simulink model "EV_assigment2"  (R2022a)
settings: Solver=VariableStepAuto  StartTime=0.0  StopTime=10800  RelTol=1e-3
libraries: spsCurrentMeasurementLib x141, spsSeriesRLCBranchLib x141, spsVoltageMeasurementLib x141, spsControlledVoltageSourceLib x140, spspowerguiLib x1
(part 3 of 15)

== system EV_assigment2/series1/Subsystem19 ==
  Controlled Voltage Source : spsControlledVoltageSourceLib/Controlled Voltage Source  Initialize=on  Source_Type=AC  Amplitude=0  Phase=0  Frequency=0  Measurements=None
  Current Measurement : spsCurrentMeasurementLib/Current Measurement  PhasorSimulation=off  OutputType=Complex  PSBequivalent=0
  Display : Display
  Display1 : Display
  Divide1 : Product  Inputs=*/
  Divide2 : Product  Inputs=*//
  Initial Capacity(Ah) : Constant  Value=28
  Integrator Limited : Integrator  LimitOutput=on  UpperSaturationLimit=1  LowerSaturationLimit=0
  LoadAh : Scope
  Product : Product
  SOC : Scope
  SOC value : Display
  Scope : Scope
  Scope1 : Scope
  Series RLC Branch : spsSeriesRLCBranchLib/Series RLC Branch  LConnTagsString=__new0  RConnTagsString=__new0  BranchType=R  Resistance=1e-6  Inductance=1e-3  SetiL0=off  InitialCurrent=0  Capacitance=1e-6  Setx0=off  InitialVoltage=0  Measurements=None
  Subsystem : Subsystem
  Subsystem1 : Subsystem
  Sum : Sum  Inputs=|+-
  Sum1 : Sum  Inputs=+--
  Voltage Measurement : spsVoltageMeasurementLib/Voltage Measurement  PhasorSimulation=off  OutputType=Complex  PSBequivalent=0
  battery Temp(k) : Constant  Value=300
  + : PMIOPort  Side=Left
  - : PMIOPort  Port=2  Side=Right
  wires:
  Subsystem/3(R1) -> Divide2/2
  Divide1/1 -> Sum/1
  Product/1 -> Sum1/2
  Current Measurement/1 -> Display1/1, Scope/1, Divide1/1, Product/2, Subsystem1/1(Battery Current)
  Subsystem/1(Em) -> Sum1/1
  battery Temp(k)/1 -> Subsystem1/3(Temp(K)), Subsystem/2(Battery temp)
  Sum/1 -> Integrator Limited/1
  Divide2/1 -> Sum/2
  Subsystem/2(R0) -> Product/1
  Integrator Limited/1 -> Divide2/1, Sum1/3
  Subsystem/4(C1) -> Divide2/3, Divide1/2
  Sum1/1 -> Controlled Voltage Source/1
  Subsystem1/2(SOC) -> Subsystem/1(SOC), SOC value/1, SOC/1
  Subsystem1/1(LoadAh) -> LoadAh/1
  Initial Capacity(Ah)/1 -> Subsystem1/2(InitCap(Ah))
  Voltage Measurement/1 -> Display/1, Scope1/1
  connections:
  Series RLC Branch/RConn1 -- Voltage Measurement/LConn1 -- Current Measurement/LConn1
  Current Measurement/RConn1 -- +/RConn1
  Controlled Voltage Source/LConn1 -- Voltage Measurement/LConn2 -- -/RConn1
  Series RLC Branch/LConn1 -- Controlled Voltage Source/RConn1

== system EV_assigment2/series1/Subsystem2 ==
  Controlled Voltage Source : spsControlledVoltageSourceLib/Controlled Voltage Source  Initialize=on  Source_Type=AC  Amplitude=0  Phase=0  Frequency=0  Measurements=None
  Current Measurement : spsCurrentMeasurementLib/Current Measurement  PhasorSimulation=off  OutputType=Complex  PSBequivalent=0
  Display : Display
  Display1 : Display
  Divide1 : Product  Inputs=*/
  Divide2 : Product  Inputs=*//
  Initial Capacity(Ah) : Constant  Value=28
  Integrator Limited : Integrator  LimitOutput=on  UpperSaturationLimit=1  LowerSaturationLimit=0
  LoadAh : Scope
  Product : Product
  SOC : Scope
  SOC value : Display
  Scope : Scope
  Scope1 : Scope
  Series RLC Branch : spsSeriesRLCBranchLib/Series RLC Branch  LConnTagsString=__new0  RConnTagsString=__new0  BranchType=R  Resistance=1e-6  Inductance=1e-3  SetiL0=off  InitialCurrent=0  Capacitance=1e-6  Setx0=off  InitialVoltage=0  Measurements=None
  Subsystem : Subsystem
  Subsystem1 : Subsystem
  Sum : Sum  Inputs=|+-
  Sum1 : Sum  Inputs=+--
  Voltage Measurement : spsVoltageMeasurementLib/Voltage Measurement  PhasorSimulation=off  OutputType=Complex  PSBequivalent=0
  battery Temp(k) : Constant  Value=300
  + : PMIOPort  Side=Left
  - : PMIOPort  Port=2  Side=Right
  wires:
  Subsystem/3(R1) -> Divide2/2
  Divide1/1 -> Sum/1
  Product/1 -> Sum1/2
  Current Measurement/1 -> Display1/1, Scope/1, Divide1/1, Product/2, Subsystem1/1(Battery Current)
  Subsystem/1(Em) -> Sum1/1
  battery Temp(k)/1 -> Subsystem1/3(Temp(K)), Subsystem/2(Battery temp)
  Sum/1 -> Integrator Limited/1
  Divide2/1 -> Sum/2
  Subsystem/2(R0) -> Product/1
  Integrator Limited/1 -> Divide2/1, Sum1/3
  Subsystem/4(C1) -> Divide2/3, Divide1/2
  Sum1/1 -> Controlled Voltage Source/1
  Subsystem1/2(SOC) -> Subsystem/1(SOC), SOC value/1, SOC/1
  Subsystem1/1(LoadAh) -> LoadAh/1
  Initial Capacity(Ah)/1 -> Subsystem1/2(InitCap(Ah))
  Voltage Measurement/1 -> Display/1, Scope1/1
  connections:
  Series RLC Branch/RConn1 -- Voltage Measurement/LConn1 -- Current Measurement/LConn1
  Current Measurement/RConn1 -- +/RConn1
  Controlled Voltage Source/LConn1 -- Voltage Measurement/LConn2 -- -/RConn1
  Series RLC Branch/LConn1 -- Controlled Voltage Source/RConn1

== system EV_assigment2/series1/Subsystem20 ==
  Controlled Voltage Source : spsControlledVoltageSourceLib/Controlled Voltage Source  Initialize=on  Source_Type=AC  Amplitude=0  Phase=0  Frequency=0  Measurements=None
  Current Measurement : spsCurrentMeasurementLib/Current Measurement  PhasorSimulation=off  OutputType=Complex  PSBequivalent=0
  Display : Display
  Display1 : Display
  Divide1 : Product  Inputs=*/
  Divide2 : Product  Inputs=*//
  Initial Capacity(Ah) : Constant  Value=28
  Integrator Limited : Integrator  LimitOutput=on  UpperSaturationLimit=1  LowerSaturationLimit=0
  LoadAh : Scope
  Product : Product
  SOC : Scope
  SOC value : Display
  Scope : Scope
  Scope1 : Scope
  Series RLC Branch : spsSeriesRLCBranchLib/Series RLC Branch  LConnTagsString=__new0  RConnTagsString=__new0  BranchType=R  Resistance=1e-6  Inductance=1e-3  SetiL0=off  InitialCurrent=0  Capacitance=1e-6  Setx0=off  InitialVoltage=0  Measurements=None
  Subsystem : Subsystem
  Subsystem1 : Subsystem
  Sum : Sum  Inputs=|+-
  Sum1 : Sum  Inputs=+--
  Voltage Measurement : spsVoltageMeasurementLib/Voltage Measurement  PhasorSimulation=off  OutputType=Complex  PSBequivalent=0
  battery Temp(k) : Constant  Value=300
  + : PMIOPort  Side=Left
  - : PMIOPort  Port=2  Side=Right
  wires:
  Subsystem/3(R1) -> Divide2/2
  Divide1/1 -> Sum/1
  Product/1 -> Sum1/2
  Current Measurement/1 -> Display1/1, Scope/1, Divide1/1, Product/2, Subsystem1/1(Battery Current)
  Subsystem/1(Em) -> Sum1/1
  battery Temp(k)/1 -> Subsystem1/3(Temp(K)), Subsystem/2(Battery temp)
  Sum/1 -> Integrator Limited/1
  Divide2/1 -> Sum/2
  Subsystem/2(R0) -> Product/1
  Integrator Limited/1 -> Divide2/1, Sum1/3
  Subsystem/4(C1) -> Divide2/3, Divide1/2
  Sum1/1 -> Controlled Voltage Source/1
  Subsystem1/2(SOC) -> Subsystem/1(SOC), SOC value/1, SOC/1
  Subsystem1/1(LoadAh) -> LoadAh/1
  Initial Capacity(Ah)/1 -> Subsystem1/2(InitCap(Ah))
  Voltage Measurement/1 -> Display/1, Scope1/1
  connections:
  Series RLC Branch/RConn1 -- Voltage Measurement/LConn1 -- Current Measurement/LConn1
  Current Measurement/RConn1 -- +/RConn1
  Controlled Voltage Source/LConn1 -- Voltage Measurement/LConn2 -- -/RConn1
  Series RLC Branch/LConn1 -- Controlled Voltage Source/RConn1

== system EV_assigment2/series1/Subsystem21 ==
  Controlled Voltage Source : spsControlledVoltageSourceLib/Controlled Voltage Source  Initialize=on  Source_Type=AC  Amplitude=0  Phase=0  Frequency=0  Measurements=None
  Current Measurement : spsCurrentMeasurementLib/Current Measurement  PhasorSimulation=off  OutputType=Complex  PSBequivalent=0
  Display : Display
  Display1 : Display
  Divide1 : Product  Inputs=*/
  Divide2 : Product  Inputs=*//
  Initial Capacity(Ah) : Constant  Value=28
  Integrator Limited : Integrator  LimitOutput=on  UpperSaturationLimit=1  LowerSaturationLimit=0
  LoadAh : Scope
  Product : Product
  SOC : Scope
  SOC value : Display
  Scope : Scope
  Scope1 : Scope
  Series RLC Branch : spsSeriesRLCBranchLib/Series RLC Branch  LConnTagsString=__new0  RConnTagsString=__new0  BranchType=R  Resistance=1e-6  Inductance=1e-3  SetiL0=off  InitialCurrent=0  Capacitance=1e-6  Setx0=off  InitialVoltage=0  Measurements=None
  Subsystem : Subsystem
  Subsystem1 : Subsystem
  Sum : Sum  Inputs=|+-
  Sum1 : Sum  Inputs=+--
  Voltage Measurement : spsVoltageMeasurementLib/Voltage Measurement  PhasorSimulation=off  OutputType=Complex  PSBequivalent=0
  battery Temp(k) : Constant  Value=300
  + : PMIOPort  Side=Left
  - : PMIOPort  Port=2  Side=Right
  wires:
  Subsystem/3(R1) -> Divide2/2
  Divide1/1 -> Sum/1
  Product/1 -> Sum1/2
  Current Measurement/1 -> Display1/1, Scope/1, Divide1/1, Product/2, Subsystem1/1(Battery Current)
  Subsystem/1(Em) -> Sum1/1
  battery Temp(k)/1 -> Subsystem1/3(Temp(K)), Subsystem/2(Battery temp)
  Sum/1 -> Integrator Limited/1
  Divide2/1 -> Sum/2
  Subsystem/2(R0) -> Product/1
  Integrator Limited/1 -> Divide2/1, Sum1/3
  Subsystem/4(C1) -> Divide2/3, Divide1/2
  Sum1/1 -> Controlled Voltage Source/1
  Subsystem1/2(SOC) -> Subsystem/1(SOC), SOC value/1, SOC/1
  Subsystem1/1(LoadAh) -> LoadAh/1
  Initial Capacity(Ah)/1 -> Subsystem1/2(InitCap(Ah))
  Voltage Measurement/1 -> Display/1, Scope1/1
  connections:
  Series RLC Branch/RConn1 -- Voltage Measurement/LConn1 -- Current Measurement/LConn1
  Current Measurement/RConn1 -- +/RConn1
  Controlled Voltage Source/LConn1 -- Voltage Measurement/LConn2 -- -/RConn1
  Series RLC Branch/LConn1 -- Controlled Voltage Source/RConn1

== system EV_assigment2/series1/Subsystem22 ==
  Controlled Voltage Source : spsControlledVoltageSourceLib/Controlled Voltage Source  Initialize=on  Source_Type=AC  Amplitude=0  Phase=0  Frequency=0  Measurements=None
  Current Measurement : spsCurrentMeasurementLib/Current Measurement  PhasorSimulation=off  OutputType=Complex  PSBequivalent=0
  Display : Display
  Display1 : Display
  Divide1 : Product  Inputs=*/
  Divide2 : Product  Inputs=*//
  Initial Capacity(Ah) : Constant  Value=28
  Integrator Limited : Integrator  LimitOutput=on  UpperSaturationLimit=1  LowerSaturationLimit=0
  LoadAh : Scope
  Product : Product
  SOC : Scope
  SOC value : Display
  Scope : Scope
  Scope1 : Scope
  Series RLC Branch : spsSeriesRLCBranchLib/Series RLC Branch  LConnTagsString=__new0  RConnTagsString=__new0  BranchType=R  Resistance=1e-6  Inductance=1e-3  SetiL0=off  InitialCurrent=0  Capacitance=1e-6  Setx0=off  InitialVoltage=0  Measurements=None
  Subsystem : Subsystem
  Subsystem1 : Subsystem
  Sum : Sum  Inputs=|+-
  Sum1 : Sum  Inputs=+--
  Voltage Measurement : spsVoltageMeasurementLib/Voltage Measurement  PhasorSimulation=off  OutputType=Complex  PSBequivalent=0
  battery Temp(k) : Constant  Value=300
  + : PMIOPort  Side=Left
  - : PMIOPort  Port=2  Side=Right
  wires:
  Subsystem/3(R1) -> Divide2/2
  Divide1/1 -> Sum/1
  Product/1 -> Sum1/2
  Current Measurement/1 -> Display1/1, Scope/1, Divide1/1, Product/2, Subsystem1/1(Battery Current)
  Subsystem/1(Em) -> Sum1/1
  battery Temp(k)/1 -> Subsystem1/3(Temp(K)), Subsystem/2(Battery temp)
  Sum/1 -> Integrator Limited/1
  Divide2/1 -> Sum/2
  Subsystem/2(R0) -> Product/1
  Integrator Limited/1 -> Divide2/1, Sum1/3
  Subsystem/4(C1) -> Divide2/3, Divide1/2
  Sum1/1 -> Controlled Voltage Source/1
  Subsystem1/2(SOC) -> Subsystem/1(SOC), SOC value/1, SOC/1
  Subsystem1/1(LoadAh) -> LoadAh/1
  Initial Capacity(Ah)/1 -> Subsystem1/2(InitCap(Ah))
  Voltage Measurement/1 -> Display/1, Scope1/1
  connections:
  Series RLC Branch/RConn1 -- Voltage Measurement/LConn1 -- Current Measurement/LConn1
  Current Measurement/RConn1 -- +/RConn1
  Controlled Voltage Source/LConn1 -- Voltage Measurement/LConn2 -- -/RConn1
  Series RLC Branch/LConn1 -- Controlled Voltage Source/RConn1

== system EV_assigment2/series1/Subsystem23 ==
  Controlled Voltage Source : spsControlledVoltageSourceLib/Controlled Voltage Source  Initialize=on  Source_Type=AC  Amplitude=0  Phase=0  Frequency=0  Measurements=None
  Current Measurement : spsCurrentMeasurementLib/Current Measurement  PhasorSimulation=off  OutputType=Complex  PSBequivalent=0
  Display : Display
  Display1 : Display
  Divide1 : Product  Inputs=*/
  Divide2 : Product  Inputs=*//
  Initial Capacity(Ah) : Constant  Value=28
  Integrator Limited : Integrator  LimitOutput=on  UpperSaturationLimit=1  LowerSaturationLimit=0
  LoadAh : Scope
  Product : Product
  SOC : Scope
  SOC value : Display
  Scope : Scope
  Scope1 : Scope
  Series RLC Branch : spsSeriesRLCBranchLib/Series RLC Branch  LConnTagsString=__new0  RConnTagsString=__new0  BranchType=R  Resistance=1e-6  Inductance=1e-3  SetiL0=off  InitialCurrent=0  Capacitance=1e-6  Setx0=off  InitialVoltage=0  Measurements=None
  Subsystem : Subsystem
  Subsystem1 : Subsystem
  Sum : Sum  Inputs=|+-
  Sum1 : Sum  Inputs=+--
  Voltage Measurement : spsVoltageMeasurementLib/Voltage Measurement  PhasorSimulation=off  OutputType=Complex  PSBequivalent=0
  battery Temp(k) : Constant  Value=300
  + : PMIOPort  Side=Left
  - : PMIOPort  Port=2  Side=Right
  wires:
  Subsystem/3(R1) -> Divide2/2
  Divide1/1 -> Sum/1
  Product/1 -> Sum1/2
  Current Measurement/1 -> Display1/1, Scope/1, Divide1/1, Product/2, Subsystem1/1(Battery Current)
  Subsystem/1(Em) -> Sum1/1
  battery Temp(k)/1 -> Subsystem1/3(Temp(K)), Subsystem/2(Battery temp)
  Sum/1 -> Integrator Limited/1
  Divide2/1 -> Sum/2
  Subsystem/2(R0) -> Product/1
  Integrator Limited/1 -> Divide2/1, Sum1/3
  Subsystem/4(C1) -> Divide2/3, Divide1/2
  Sum1/1 -> Controlled Voltage Source/1
  Subsystem1/2(SOC) -> Subsystem/1(SOC), SOC value/1, SOC/1
  Subsystem1/1(LoadAh) -> LoadAh/1
  Initial Capacity(Ah)/1 -> Subsystem1/2(InitCap(Ah))
  Voltage Measurement/1 -> Display/1, Scope1/1
  connections:
  Series RLC Branch/RConn1 -- Voltage Measurement/LConn1 -- Current Measurement/LConn1
  Current Measurement/RConn1 -- +/RConn1
  Controlled Voltage Source/LConn1 -- Voltage Measurement/LConn2 -- -/RConn1
  Series RLC Branch/LConn1 -- Controlled Voltage Source/RConn1

== system EV_assigment2/series1/Subsystem24 ==
  Controlled Voltage Source : spsControlledVoltageSourceLib/Controlled Voltage Source  Initialize=on  Source_Type=AC  Amplitude=0  Phase=0  Frequency=0  Measurements=None
  Current Measurement : spsCurrentMeasurementLib/Current Measurement  PhasorSimulation=off  OutputType=Complex  PSBequivalent=0
  Display : Display
  Display1 : Display
  Divide1 : Product  Inputs=*/
  Divide2 : Product  Inputs=*//
  Initial Capacity(Ah) : Constant  Value=28
  Integrator Limited : Integrator  LimitOutput=on  UpperSaturationLimit=1  LowerSaturationLimit=0
  LoadAh : Scope
  Product : Product
  SOC : Scope
  SOC value : Display
  Scope : Scope
  Scope1 : Scope
  Series RLC Branch : spsSeriesRLCBranchLib/Series RLC Branch  LConnTagsString=__new0  RConnTagsString=__new0  BranchType=R  Resistance=1e-6  Inductance=1e-3  SetiL0=off  InitialCurrent=0  Capacitance=1e-6  Setx0=off  InitialVoltage=0  Measurements=None
  Subsystem : Subsystem
  Subsystem1 : Subsystem
  Sum : Sum  Inputs=|+-
  Sum1 : Sum  Inputs=+--
  Voltage Measurement : spsVoltageMeasurementLib/Voltage Measurement  PhasorSimulation=off  OutputType=Complex  PSBequivalent=0
  battery Temp(k) : Constant  Value=300
  + : PMIOPort  Side=Left
  - : PMIOPort  Port=2  Side=Right
  wires:
  Subsystem/3(R1) -> Divide2/2
  Divide1/1 -> Sum/1
  Product/1 -> Sum1/2
  Current Measurement/1 -> Display1/1, Scope/1, Divide1/1, Product/2, Subsystem1/1(Battery Current)
  Subsystem/1(Em) -> Sum1/1
  battery Temp(k)/1 -> Subsystem1/3(Temp(K)), Subsystem/2(Battery temp)
  Sum/1 -> Integrator Limited/1
  Divide2/1 -> Sum/2
  Subsystem/2(R0) -> Product/1
  Integrator Limited/1 -> Divide2/1, Sum1/3
  Subsystem/4(C1) -> Divide2/3, Divide1/2
  Sum1/1 -> Controlled Voltage Source/1
  Subsystem1/2(SOC) -> Subsystem/1(SOC), SOC value/1, SOC/1
  Subsystem1/1(LoadAh) -> LoadAh/1
  Initial Capacity(Ah)/1 -> Subsystem1/2(InitCap(Ah))
  Voltage Measurement/1 -> Display/1, Scope1/1
  connections:
  Series RLC Branch/RConn1 -- Voltage Measurement/LConn1 -- Current Measurement/LConn1
  Current Measurement/RConn1 -- +/RConn1
  Controlled Voltage Source/LConn1 -- Voltage Measurement/LConn2 -- -/RConn1
  Series RLC Branch/LConn1 -- Controlled Voltage Source/RConn1

== system EV_assigment2/series1/Subsystem25 ==
  Controlled Voltage Source : spsControlledVoltageSourceLib/Controlled Voltage Source  Initialize=on  Source_Type=AC  Amplitude=0  Phase=0  Frequency=0  Measurements=None
  Current Measurement : spsCurrentMeasurementLib/Current Measurement  PhasorSimulation=off  OutputType=Complex  PSBequivalent=0
  Display : Display
  Display1 : Display
  Divide1 : Product  Inputs=*/
  Divide2 : Product  Inputs=*//
  Initial Capacity(Ah) : Constant  Value=28
  Integrator Limited : Integrator  LimitOutput=on  UpperSaturationLimit=1  LowerSaturationLimit=0
  LoadAh : Scope
  Product : Product
  SOC : Scope
  SOC value : Display
  Scope : Scope
  Scope1 : Scope
  Series RLC Branch : spsSeriesRLCBranchLib/Series RLC Branch  LConnTagsString=__new0  RConnTagsString=__new0  BranchType=R  Resistance=1e-6  Inductance=1e-3  SetiL0=off  InitialCurrent=0  Capacitance=1e-6  Setx0=off  InitialVoltage=0  Measurements=None
  Subsystem : Subsystem
  Subsystem1 : Subsystem
  Sum : Sum  Inputs=|+-
  Sum1 : Sum  Inputs=+--
  Voltage Measurement : spsVoltageMeasurementLib/Voltage Measurement  PhasorSimulation=off  OutputType=Complex  PSBequivalent=0
  battery Temp(k) : Constant  Value=300
  + : PMIOPort  Side=Left
  - : PMIOPort  Port=2  Side=Right
  wires:
  Subsystem/3(R1) -> Divide2/2
  Divide1/1 -> Sum/1
  Product/1 -> Sum1/2
  Current Measurement/1 -> Display1/1, Scope/1, Divide1/1, Product/2, Subsystem1/1(Battery Current)
  Subsystem/1(Em) -> Sum1/1
  battery Temp(k)/1 -> Subsystem1/3(Temp(K)), Subsystem/2(Battery temp)
  Sum/1 -> Integrator Limited/1
  Divide2/1 -> Sum/2
  Subsystem/2(R0) -> Product/1
  Integrator Limited/1 -> Divide2/1, Sum1/3
  Subsystem/4(C1) -> Divide2/3, Divide1/2
  Sum1/1 -> Controlled Voltage Source/1
  Subsystem1/2(SOC) -> Subsystem/1(SOC), SOC value/1, SOC/1
  Subsystem1/1(LoadAh) -> LoadAh/1
  Initial Capacity(Ah)/1 -> Subsystem1/2(InitCap(Ah))
  Voltage Measurement/1 -> Display/1, Scope1/1
  connections:
  Series RLC Branch/RConn1 -- Voltage Measurement/LConn1 -- Current Measurement/LConn1
  Current Measurement/RConn1 -- +/RConn1
  Controlled Voltage Source/LConn1 -- Voltage Measurement/LConn2 -- -/RConn1
  Series RLC Branch/LConn1 -- Controlled Voltage Source/RConn1

== system EV_assigment2/series1/Subsystem26 ==
  Controlled Voltage Source : spsControlledVoltageSourceLib/Controlled Voltage Source  Initialize=on  Source_Type=AC  Amplitude=0  Phase=0  Frequency=0  Measurements=None
  Current Measurement : spsCurrentMeasurementLib/Current Measurement  PhasorSimulation=off  OutputType=Complex  PSBequivalent=0
  Display : Display
  Display1 : Display
  Divide1 : Product  Inputs=*/
  Divide2 : Product  Inputs=*//
  Initial Capacity(Ah) : Constant  Value=28
  Integrator Limited : Integrator  LimitOutput=on  UpperSaturationLimit=1  LowerSaturationLimit=0
  LoadAh : Scope
  Product : Product
  SOC : Scope
  SOC value : Display
  Scope : Scope
  Scope1 : Scope
  Series RLC Branch : spsSeriesRLCBranchLib/Series RLC Branch  LConnTagsString=__new0  RConnTagsString=__new0  BranchType=R  Resistance=1e-6  Inductance=1e-3  SetiL0=off  InitialCurrent=0  Capacitance=1e-6  Setx0=off  InitialVoltage=0  Measurements=None
  Subsystem : Subsystem
  Subsystem1 : Subsystem
  Sum : Sum  Inputs=|+-
  Sum1 : Sum  Inputs=+--
  Voltage Measurement : spsVoltageMeasurementLib/Voltage Measurement  PhasorSimulation=off  OutputType=Complex  PSBequivalent=0
  battery Temp(k) : Constant  Value=300
  + : PMIOPort  Side=Left
  - : PMIOPort  Port=2  Side=Right
  wires:
  Subsystem/3(R1) -> Divide2/2
  Divide1/1 -> Sum/1
  Product/1 -> Sum1/2
  Current Measurement/1 -> Display1/1, Scope/1, Divide1/1, Product/2, Subsystem1/1(Battery Current)
  Subsystem/1(Em) -> Sum1/1
  battery Temp(k)/1 -> Subsystem1/3(Temp(K)), Subsystem/2(Battery temp)
  Sum/1 -> Integrator Limited/1
  Divide2/1 -> Sum/2
  Subsystem/2(R0) -> Product/1
  Integrator Limited/1 -> Divide2/1, Sum1/3
  Subsystem/4(C1) -> Divide2/3, Divide1/2
  Sum1/1 -> Controlled Voltage Source/1
  Subsystem1/2(SOC) -> Subsystem/1(SOC), SOC value/1, SOC/1
  Subsystem1/1(LoadAh) -> LoadAh/1
  Initial Capacity(Ah)/1 -> Subsystem1/2(InitCap(Ah))
  Voltage Measurement/1 -> Display/1, Scope1/1
  connections:
  Series RLC Branch/RConn1 -- Voltage Measurement/LConn1 -- Current Measurement/LConn1
  Current Measurement/RConn1 -- +/RConn1
  Controlled Voltage Source/LConn1 -- Voltage Measurement/LConn2 -- -/RConn1
  Series RLC Branch/LConn1 -- Controlled Voltage Source/RConn1

== system EV_assigment2/series1/Subsystem27 ==
  Controlled Voltage Source : spsControlledVoltageSourceLib/Controlled Voltage Source  Initialize=on  Source_Type=AC  Amplitude=0  Phase=0  Frequency=0  Measurements=None
  Current Measurement : spsCurrentMeasurementLib/Current Measurement  PhasorSimulation=off  OutputType=Complex  PSBequivalent=0
  Display : Display
  Display1 : Display
  Divide1 : Product  Inputs=*/
  Divide2 : Product  Inputs=*//
  Initial Capacity(Ah) : Constant  Value=28
  Integrator Limited : Integrator  LimitOutput=on  UpperSaturationLimit=1  LowerSaturationLimit=0
  LoadAh : Scope
  Product : Product
  SOC : Scope
  SOC value : Display
  Scope : Scope
  Scope1 : Scope
  Series RLC Branch : spsSeriesRLCBranchLib/Series RLC Branch  LConnTagsString=__new0  RConnTagsString=__new0  BranchType=R  Resistance=1e-6  Inductance=1e-3  SetiL0=off  InitialCurrent=0  Capacitance=1e-6  Setx0=off  InitialVoltage=0  Measurements=None
  Subsystem : Subsystem
  Subsystem1 : Subsystem
  Sum : Sum  Inputs=|+-
  Sum1 : Sum  Inputs=+--
  Voltage Measurement : spsVoltageMeasurementLib/Voltage Measurement  PhasorSimulation=off  OutputType=Complex  PSBequivalent=0
  battery Temp(k) : Constant  Value=300
  + : PMIOPort  Side=Left
  - : PMIOPort  Port=2  Side=Right
  wires:
  Subsystem/3(R1) -> Divide2/2
  Divide1/1 -> Sum/1
  Product/1 -> Sum1/2
  Current Measurement/1 -> Display1/1, Scope/1, Divide1/1, Product/2, Subsystem1/1(Battery Current)
  Subsystem/1(Em) -> Sum1/1
  battery Temp(k)/1 -> Subsystem1/3(Temp(K)), Subsystem/2(Battery temp)
  Sum/1 -> Integrator Limited/1
  Divide2/1 -> Sum/2
  Subsystem/2(R0) -> Product/1
  Integrator Limited/1 -> Divide2/1, Sum1/3
  Subsystem/4(C1) -> Divide2/3, Divide1/2
  Sum1/1 -> Controlled Voltage Source/1
  Subsystem1/2(SOC) -> Subsystem/1(SOC), SOC value/1, SOC/1
  Subsystem1/1(LoadAh) -> LoadAh/1
  Initial Capacity(Ah)/1 -> Subsystem1/2(InitCap(Ah))
  Voltage Measurement/1 -> Display/1, Scope1/1
  connections:
  Series RLC Branch/RConn1 -- Voltage Measurement/LConn1 -- Current Measurement/LConn1
  Current Measurement/RConn1 -- +/RConn1
  Controlled Voltage Source/LConn1 -- Voltage Measurement/LConn2 -- -/RConn1
  Series RLC Branch/LConn1 -- Controlled Voltage Source/RConn1

== system EV_assigment2/series1/Subsystem28 ==
  Controlled Voltage Source : spsControlledVoltageSourceLib/Controlled Voltage Source  Initialize=on  Source_Type=AC  Amplitude=0  Phase=0  Frequency=0  Measurements=None
  Current Measurement : spsCurrentMeasurementLib/Current Measurement  PhasorSimulation=off  OutputType=Complex  PSBequivalent=0
  Display : Display
  Display1 : Display
  Divide1 : Product  Inputs=*/
  Divide2 : Product  Inputs=*//
  Initial Capacity(Ah) : Constant  Value=28
  Integrator Limited : Integrator  LimitOutput=on  UpperSaturationLimit=1  LowerSaturationLimit=0
  LoadAh : Scope
  Product : Product
  SOC : Scope
  SOC value : Display
  Scope : Scope
  Scope1 : Scope
  Series RLC Branch : spsSeriesRLCBranchLib/Series RLC Branch  LConnTagsString=__new0  RConnTagsString=__new0  BranchType=R  Resistance=1e-6  Inductance=1e-3  SetiL0=off  InitialCurrent=0  Capacitance=1e-6  Setx0=off  InitialVoltage=0  Measurements=None
  Subsystem : Subsystem
  Subsystem1 : Subsystem
  Sum : Sum  Inputs=|+-
  Sum1 : Sum  Inputs=+--
  Voltage Measurement : spsVoltageMeasurementLib/Voltage Measurement  PhasorSimulation=off  OutputType=Complex  PSBequivalent=0
  battery Temp(k) : Constant  Value=300
  + : PMIOPort  Side=Left
  - : PMIOPort  Port=2  Side=Right
  wires:
  Subsystem/3(R1) -> Divide2/2
  Divide1/1 -> Sum/1
  Product/1 -> Sum1/2
  Current Measurement/1 -> Display1/1, Scope/1, Divide1/1, Product/2, Subsystem1/1(Battery Current)
  Subsystem/1(Em) -> Sum1/1
  battery Temp(k)/1 -> Subsystem1/3(Temp(K)), Subsystem/2(Battery temp)
  Sum/1 -> Integrator Limited/1
  Divide2/1 -> Sum/2
  Subsystem/2(R0) -> Product/1
  Integrator Limited/1 -> Divide2/1, Sum1/3
  Subsystem/4(C1) -> Divide2/3, Divide1/2
  Sum1/1 -> Controlled Voltage Source/1
  Subsystem1/2(SOC) -> Subsystem/1(SOC), SOC value/1, SOC/1
  Subsystem1/1(LoadAh) -> LoadAh/1
  Initial Capacity(Ah)/1 -> Subsystem1/2(InitCap(Ah))
  Voltage Measurement/1 -> Display/1, Scope1/1
  connections:
  Series RLC Branch/RConn1 -- Voltage Measurement/LConn1 -- Current Measurement/LConn1
  Current Measurement/RConn1 -- +/RConn1
  Controlled Voltage Source/LConn1 -- Voltage Measurement/LConn2 -- -/RConn1
  Series RLC Branch/LConn1 -- Controlled Voltage Source/RConn1

== system EV_assigment2/series1/Subsystem3 ==
  Controlled Voltage Source : spsControlledVoltageSourceLib/Controlled Voltage Source  Initialize=on  Source_Type=AC  Amplitude=0  Phase=0  Frequency=0  Measurements=None
  Current Measurement : spsCurrentMeasurementLib/Current Measurement  PhasorSimulation=off  OutputType=Complex  PSBequivalent=0
  Display : Display
  Display1 : Display
  Divide1 : Product  Inputs=*/
  Divide2 : Product  Inputs=*//
  Initial Capacity(Ah) : Constant  Value=28
  Integrator Limited : Integrator  LimitOutput=on  UpperSaturationLimit=1  LowerSaturationLimit=0
  LoadAh : Scope
  Product : Product
  SOC : Scope
  SOC value : Display
  Scope : Scope
  Scope1 : Scope
  Series RLC Branch : spsSeriesRLCBranchLib/Series RLC Branch  LConnTagsString=__new0  RConnTagsString=__new0  BranchType=R  Resistance=1e-6  Inductance=1e-3  SetiL0=off  InitialCurrent=0  Capacitance=1e-6  Setx0=off  InitialVoltage=0  Measurements=None
  Subsystem : Subsystem
  Subsystem1 : Subsystem
  Sum : Sum  Inputs=|+-
  Sum1 : Sum  Inputs=+--
  Voltage Measurement : spsVoltageMeasurementLib/Voltage Measurement  PhasorSimulation=off  OutputType=Complex  PSBequivalent=0
  battery Temp(k) : Constant  Value=300
  + : PMIOPort  Side=Left
  - : PMIOPort  Port=2  Side=Right
  wires:
  Subsystem/3(R1) -> Divide2/2
  Divide1/1 -> Sum/1
  Product/1 -> Sum1/2
  Current Measurement/1 -> Display1/1, Scope/1, Divide1/1, Product/2, Subsystem1/1(Battery Current)
  Subsystem/1(Em) -> Sum1/1
  battery Temp(k)/1 -> Subsystem1/3(Temp(K)), Subsystem/2(Battery temp)
  Sum/1 -> Integrator Limited/1
  Divide2/1 -> Sum/2
  Subsystem/2(R0) -> Product/1
  Integrator Limited/1 -> Divide2/1, Sum1/3
  Subsystem/4(C1) -> Divide2/3, Divide1/2
  Sum1/1 -> Controlled Voltage Source/1
  Subsystem1/2(SOC) -> Subsystem/1(SOC), SOC value/1, SOC/1
  Subsystem1/1(LoadAh) -> LoadAh/1
  Initial Capacity(Ah)/1 -> Subsystem1/2(InitCap(Ah))
  Voltage Measurement/1 -> Display/1, Scope1/1
  connections:
  Series RLC Branch/RConn1 -- Voltage Measurement/LConn1 -- Current Measurement/LConn1
  Current Measurement/RConn1 -- +/RConn1
  Controlled Voltage Source/LConn1 -- Voltage Measurement/LConn2 -- -/RConn1
  Series RLC Branch/LConn1 -- Controlled Voltage Source/RConn1

== system EV_assigment2/series1/Subsystem4 ==
  Controlled Voltage Source : spsControlledVoltageSourceLib/Controlled Voltage Source  Initialize=on  Source_Type=AC  Amplitude=0  Phase=0  Frequency=0  Measurements=None
  Current Measurement : spsCurrentMeasurementLib/Current Measurement  PhasorSimulation=off  OutputType=Complex  PSBequivalent=0
  Display : Display
  Display1 : Display
  Divide1 : Product  Inputs=*/
  Divide2 : Product  Inputs=*//
  Initial Capacity(Ah) : Constant  Value=28
  Integrator Limited : Integrator  LimitOutput=on  UpperSaturationLimit=1  LowerSaturationLimit=0
  LoadAh : Scope
  Product : Product
  SOC : Scope
  SOC value : Display
  Scope : Scope
  Scope1 : Scope
  Series RLC Branch : spsSeriesRLCBranchLib/Series RLC Branch  LConnTagsString=__new0  RConnTagsString=__new0  BranchType=R  Resistance=1e-6  Inductance=1e-3  SetiL0=off  InitialCurrent=0  Capacitance=1e-6  Setx0=off  InitialVoltage=0  Measurements=None
  Subsystem : Subsystem
  Subsystem1 : Subsystem
  Sum : Sum  Inputs=|+-
  Sum1 : Sum  Inputs=+--
  Voltage Measurement : spsVoltageMeasurementLib/Voltage Measurement  PhasorSimulation=off  OutputType=Complex  PSBequivalent=0
  battery Temp(k) : Constant  Value=300
  + : PMIOPort  Side=Left
  - : PMIOPort  Port=2  Side=Right
  wires:
  Subsystem/3(R1) -> Divide2/2
  Divide1/1 -> Sum/1
  Product/1 -> Sum1/2
  Current Measurement/1 -> Display1/1, Scope/1, Divide1/1, Product/2, Subsystem1/1(Battery Current)
  Subsystem/1(Em) -> Sum1/1
  battery Temp(k)/1 -> Subsystem1/3(Temp(K)), Subsystem/2(Battery temp)
  Sum/1 -> Integrator Limited/1
  Divide2/1 -> Sum/2
  Subsystem/2(R0) -> Product/1
  Integrator Limited/1 -> Divide2/1, Sum1/3
  Subsystem/4(C1) -> Divide2/3, Divide1/2
  Sum1/1 -> Controlled Voltage Source/1
  Subsystem1/2(SOC) -> Subsystem/1(SOC), SOC value/1, SOC/1
  Subsystem1/1(LoadAh) -> LoadAh/1
  Initial Capacity(Ah)/1 -> Subsystem1/2(InitCap(Ah))
  Voltage Measurement/1 -> Display/1, Scope1/1
  connections:
  Series RLC Branch/RConn1 -- Voltage Measurement/LConn1 -- Current Measurement/LConn1
  Current Measurement/RConn1 -- +/RConn1
  Controlled Voltage Source/LConn1 -- Voltage Measurement/LConn2 -- -/RConn1
  Series RLC Branch/LConn1 -- Controlled Voltage Source/RConn1

== system EV_assigment2/series1/Subsystem5 ==
  Controlled Voltage Source : spsControlledVoltageSourceLib/Controlled Voltage Source  Initialize=on  Source_Type=AC  Amplitude=0  Phase=0  Frequency=0  Measurements=None
  Current Measurement : spsCurrentMeasurementLib/Current Measurement  PhasorSimulation=off  OutputType=Complex  PSBequivalent=0
  Display : Display
  Display1 : Display
  Divide1 : Product  Inputs=*/
  Divide2 : Product  Inputs=*//
  Initial Capacity(Ah) : Constant  Value=28
  Integrator Limited : Integrator  LimitOutput=on  UpperSaturationLimit=1  LowerSaturationLimit=0
  LoadAh : Scope
  Product : Product
  SOC : Scope
  SOC value : Display
  Scope : Scope
  Scope1 : Scope
  Series RLC Branch : spsSeriesRLCBranchLib/Series RLC Branch  LConnTagsString=__new0  RConnTagsString=__new0  BranchType=R  Resistance=1e-6  Inductance=1e-3  SetiL0=off  InitialCurrent=0  Capacitance=1e-6  Setx0=off  InitialVoltage=0  Measurements=None
  Subsystem : Subsystem
  Subsystem1 : Subsystem
  Sum : Sum  Inputs=|+-
  Sum1 : Sum  Inputs=+--
  Voltage Measurement : spsVoltageMeasurementLib/Voltage Measurement  PhasorSimulation=off  OutputType=Complex  PSBequivalent=0
  battery Temp(k) : Constant  Value=300
  + : PMIOPort  Side=Left
  - : PMIOPort  Port=2  Side=Right
  wires:
  Subsystem/3(R1) -> Divide2/2
  Divide1/1 -> Sum/1
  Product/1 -> Sum1/2
  Current Measurement/1 -> Display1/1, Scope/1, Divide1/1, Product/2, Subsystem1/1(Battery Current)
  Subsystem/1(Em) -> Sum1/1
  battery Temp(k)/1 -> Subsystem1/3(Temp(K)), Subsystem/2(Battery temp)
  Sum/1 -> Integrator Limited/1
  Divide2/1 -> Sum/2
  Subsystem/2(R0) -> Product/1
  Integrator Limited/1 -> Divide2/1, Sum1/3
  Subsystem/4(C1) -> Divide2/3, Divide1/2
  Sum1/1 -> Controlled Voltage Source/1
  Subsystem1/2(SOC) -> Subsystem/1(SOC), SOC value/1, SOC/1
  Subsystem1/1(LoadAh) -> LoadAh/1
  Initial Capacity(Ah)/1 -> Subsystem1/2(InitCap(Ah))
  Voltage Measurement/1 -> Display/1, Scope1/1
  connections:
  Series RLC Branch/RConn1 -- Voltage Measurement/LConn1 -- Current Measurement/LConn1
  Current Measurement/RConn1 -- +/RConn1
  Controlled Voltage Source/LConn1 -- Voltage Measurement/LConn2 -- -/RConn1
  Series RLC Branch/LConn1 -- Controlled Voltage Source/RConn1

== system EV_assigment2/series1/Subsystem6 ==
  Controlled Voltage Source : spsControlledVoltageSourceLib/Controlled Voltage Source  Initialize=on  Source_Type=AC  Amplitude=0  Phase=0  Frequency=0  Measurements=None
  Current Measurement : spsCurrentMeasurementLib/Current Measurement  PhasorSimulation=off  OutputType=Complex  PSBequivalent=0
  Display : Display
  Display1 : Display
  Divide1 : Product  Inputs=*/
  Divide2 : Product  Inputs=*//
  Initial Capacity(Ah) : Constant  Value=28
  Integrator Limited : Integrator  LimitOutput=on  UpperSaturationLimit=1  LowerSaturationLimit=0
  LoadAh : Scope
  Product : Product
  SOC : Scope
  SOC value : Display
  Scope : Scope
  Scope1 : Scope
  Series RLC Branch : spsSeriesRLCBranchLib/Series RLC Branch  LConnTagsString=__new0  RConnTagsString=__new0  BranchType=R  Resistance=1e-6  Inductance=1e-3  SetiL0=off  InitialCurrent=0  Capacitance=1e-6  Setx0=off  InitialVoltage=0  Measurements=None
  Subsystem : Subsystem
  Subsystem1 : Subsystem
  Sum : Sum  Inputs=|+-
  Sum1 : Sum  Inputs=+--
  Voltage Measurement : spsVoltageMeasurementLib/Voltage Measurement  PhasorSimulation=off  OutputType=Complex  PSBequivalent=0
  battery Temp(k) : Constant  Value=300
  + : PMIOPort  Side=Left
  - : PMIOPort  Port=2  Side=Right
  wires:
  Subsystem/3(R1) -> Divide2/2
  Divide1/1 -> Sum/1
  Product/1 -> Sum1/2
  Current Measurement/1 -> Display1/1, Scope/1, Divide1/1, Product/2, Subsystem1/1(Battery Current)
  Subsystem/1(Em) -> Sum1/1
  battery Temp(k)/1 -> Subsystem1/3(Temp(K)), Subsystem/2(Battery temp)
  Sum/1 -> Integrator Limited/1
  Divide2/1 -> Sum/2
  Subsystem/2(R0) -> Product/1
  Integrator Limited/1 -> Divide2/1, Sum1/3
  Subsystem/4(C1) -> Divide2/3, Divide1/2
  Sum1/1 -> Controlled Voltage Source/1
  Subsystem1/2(SOC) -> Subsystem/1(SOC), SOC value/1, SOC/1
  Subsystem1/1(LoadAh) -> LoadAh/1
  Initial Capacity(Ah)/1 -> Subsystem1/2(InitCap(Ah))
  Voltage Measurement/1 -> Display/1, Scope1/1
  connections:
  Series RLC Branch/RConn1 -- Voltage Measurement/LConn1 -- Current Measurement/LConn1
  Current Measurement/RConn1 -- +/RConn1
  Controlled Voltage Source/LConn1 -- Voltage Measurement/LConn2 -- -/RConn1
  Series RLC Branch/LConn1 -- Controlled Voltage Source/RConn1

== system EV_assigment2/series1/Subsystem7 ==
  Controlled Voltage Source : spsControlledVoltageSourceLib/Controlled Voltage Source  Initialize=on  Source_Type=AC  Amplitude=0  Phase=0  Frequency=0  Measurements=None
  Current Measurement : spsCurrentMeasurementLib/Current Measurement  PhasorSimulation=off  OutputType=Complex  PSBequivalent=0
  Display : Display
  Display1 : Display
  Divide1 : Product  Inputs=*/
  Divide2 : Product  Inputs=*//
  Initial Capacity(Ah) : Constant  Value=28
  Integrator Limited : Integrator  LimitOutput=on  UpperSaturationLimit=1  LowerSaturationLimit=0
  LoadAh : Scope
  Product : Product
  SOC : Scope
  SOC value : Display
  Scope : Scope
  Scope1 : Scope
  Series RLC Branch : spsSeriesRLCBranchLib/Series RLC Branch  LConnTagsString=__new0  RConnTagsString=__new0  BranchType=R  Resistance=1e-6  Inductance=1e-3  SetiL0=off  InitialCurrent=0  Capacitance=1e-6  Setx0=off  InitialVoltage=0  Measurements=None
  Subsystem : Subsystem
  Subsystem1 : Subsystem
  Sum : Sum  Inputs=|+-
  Sum1 : Sum  Inputs=+--
  Voltage Measurement : spsVoltageMeasurementLib/Voltage Measurement  PhasorSimulation=off  OutputType=Complex  PSBequivalent=0
  battery Temp(k) : Constant  Value=300
  + : PMIOPort  Side=Left
  - : PMIOPort  Port=2  Side=Right
  wires:
  Subsystem/3(R1) -> Divide2/2
  Divide1/1 -> Sum/1
  Product/1 -> Sum1/2
  Current Measurement/1 -> Display1/1, Scope/1, Divide1/1, Product/2, Subsystem1/1(Battery Current)
  Subsystem/1(Em) -> Sum1/1
  battery Temp(k)/1 -> Subsystem1/3(Temp(K)), Subsystem/2(Battery temp)
  Sum/1 -> Integrator Limited/1
  Divide2/1 -> Sum/2
  Subsystem/2(R0) -> Product/1
  Integrator Limited/1 -> Divide2/1, Sum1/3
  Subsystem/4(C1) -> Divide2/3, Divide1/2
  Sum1/1 -> Controlled Voltage Source/1
  Subsystem1/2(SOC) -> Subsystem/1(SOC), SOC value/1, SOC/1
  Subsystem1/1(LoadAh) -> LoadAh/1
  Initial Capacity(Ah)/1 -> Subsystem1/2(InitCap(Ah))
  Voltage Measurement/1 -> Display/1, Scope1/1
  connections:
  Series RLC Branch/RConn1 -- Voltage Measurement/LConn1 -- Current Measurement/LConn1
  Current Measurement/RConn1 -- +/RConn1
  Controlled Voltage Source/LConn1 -- Voltage Measurement/LConn2 -- -/RConn1
  Series RLC Branch/LConn1 -- Controlled Voltage Source/RConn1

== system EV_assigment2/series1/Subsystem8 ==
  Controlled Voltage Source : spsControlledVoltageSourceLib/Controlled Voltage Source  Initialize=on  Source_Type=AC  Amplitude=0  Phase=0  Frequency=0  Measurements=None
  Current Measurement : spsCurrentMeasurementLib/Current Measurement  PhasorSimulation=off  OutputType=Complex  PSBequivalent=0
  Display : Display
  Display1 : Display
  Divide1 : Product  Inputs=*/
  Divide2 : Product  Inputs=*//
  Initial Capacity(Ah) : Constant  Value=28
  Integrator Limited : Integrator  LimitOutput=on  UpperSaturationLimit=1  LowerSaturationLimit=0
  LoadAh : Scope
  Product : Product
  SOC : Scope
  SOC value : Display
  Scope : Scope
  Scope1 : Scope
  Series RLC Branch : spsSeriesRLCBranchLib/Series RLC Branch  LConnTagsString=__new0  RConnTagsString=__new0  BranchType=R  Resistance=1e-6  Inductance=1e-3  SetiL0=off  InitialCurrent=0  Capacitance=1e-6  Setx0=off  InitialVoltage=0  Measurements=None
  Subsystem : Subsystem
  Subsystem1 : Subsystem
  Sum : Sum  Inputs=|+-
  Sum1 : Sum  Inputs=+--
  Voltage Measurement : spsVoltageMeasurementLib/Voltage Measurement  PhasorSimulation=off  OutputType=Complex  PSBequivalent=0
  battery Temp(k) : Constant  Value=300
  + : PMIOPort  Side=Left
  - : PMIOPort  Port=2  Side=Right
  wires:
  Subsystem/3(R1) -> Divide2/2
  Divide1/1 -> Sum/1
  Product/1 -> Sum1/2
  Current Measurement/1 -> Display1/1, Scope/1, Divide1/1, Product/2, Subsystem1/1(Battery Current)
  Subsystem/1(Em) -> Sum1/1
  battery Temp(k)/1 -> Subsystem1/3(Temp(K)), Subsystem/2(Battery temp)
  Sum/1 -> Integrator Limited/1
  Divide2/1 -> Sum/2
  Subsystem/2(R0) -> Product/1
  Integrator Limited/1 -> Divide2/1, Sum1/3
  Subsystem/4(C1) -> Divide2/3, Divide1/2
  Sum1/1 -> Controlled Voltage Source/1
  Subsystem1/2(SOC) -> Subsystem/1(SOC), SOC value/1, SOC/1
  Subsystem1/1(LoadAh) -> LoadAh/1
  Initial Capacity(Ah)/1 -> Subsystem1/2(InitCap(Ah))
  Voltage Measurement/1 -> Display/1, Scope1/1
  connections:
  Series RLC Branch/RConn1 -- Voltage Measurement/LConn1 -- Current Measurement/LConn1
  Current Measurement/RConn1 -- +/RConn1
  Controlled Voltage Source/LConn1 -- Voltage Measurement/LConn2 -- -/RConn1
  Series RLC Branch/LConn1 -- Controlled Voltage Source/RConn1

== system EV_assigment2/series1/Subsystem9 ==
  Controlled Voltage Source : spsControlledVoltageSourceLib/Controlled Voltage Source  Initialize=on  Source_Type=AC  Amplitude=0  Phase=0  Frequency=0  Measurements=None
  Current Measurement : spsCurrentMeasurementLib/Current Measurement  PhasorSimulation=off  OutputType=Complex  PSBequivalent=0
  Display : Display
  Display1 : Display
  Divide1 : Product  Inputs=*/
  Divide2 : Product  Inputs=*//
  Initial Capacity(Ah) : Constant  Value=28
  Integrator Limited : Integrator  LimitOutput=on  UpperSaturationLimit=1  LowerSaturationLimit=0
  LoadAh : Scope
  Product : Product
  SOC : Scope
  SOC value : Display
  Scope : Scope
  Scope1 : Scope
  Series RLC Branch : spsSeriesRLCBranchLib/Series RLC Branch  LConnTagsString=__new0  RConnTagsString=__new0  BranchType=R  Resistance=1e-6  Inductance=1e-3  SetiL0=off  InitialCurrent=0  Capacitance=1e-6  Setx0=off  InitialVoltage=0  Measurements=None
  Subsystem : Subsystem
  Subsystem1 : Subsystem
  Sum : Sum  Inputs=|+-
  Sum1 : Sum  Inputs=+--
  Voltage Measurement : spsVoltageMeasurementLib/Voltage Measurement  PhasorSimulation=off  OutputType=Complex  PSBequivalent=0
  battery Temp(k) : Constant  Value=300
  + : PMIOPort  Side=Left
  - : PMIOPort  Port=2  Side=Right
  wires:
  Subsystem/3(R1) -> Divide2/2
  Divide1/1 -> Sum/1
  Product/1 -> Sum1/2
  Current Measurement/1 -> Display1/1, Scope/1, Divide1/1, Product/2, Subsystem1/1(Battery Current)
  Subsystem/1(Em) -> Sum1/1
  battery Temp(k)/1 -> Subsystem1/3(Temp(K)), Subsystem/2(Battery temp)
  Sum/1 -> Integrator Limited/1
  Divide2/1 -> Sum/2
  Subsystem/2(R0) -> Product/1
  Integrator Limited/1 -> Divide2/1, Sum1/3
  Subsystem/4(C1) -> Divide2/3, Divide1/2
  Sum1/1 -> Controlled Voltage Source/1
  Subsystem1/2(SOC) -> Subsystem/1(SOC), SOC value/1, SOC/1
  Subsystem1/1(LoadAh) -> LoadAh/1
  Initial Capacity(Ah)/1 -> Subsystem1/2(InitCap(Ah))
  Voltage Measurement/1 -> Display/1, Scope1/1
  connections:
  Series RLC Branch/RConn1 -- Voltage Measurement/LConn1 -- Current Measurement/LConn1
  Current Measurement/RConn1 -- +/RConn1
  Controlled Voltage Source/LConn1 -- Voltage Measurement/LConn2 -- -/RConn1
  Series RLC Branch/LConn1 -- Controlled Voltage Source/RConn1

== system EV_assigment2/series2/Subsystem1 ==
  Controlled Voltage Source : spsControlledVoltageSourceLib/Controlled Voltage Source  Initialize=on  Source_Type=AC  Amplitude=0  Phase=0  Frequency=0  Measurements=None
  Current Measurement : spsCurrentMeasurementLib/Current Measurement  PhasorSimulation=off  OutputType=Complex  PSBequivalent=0
  Display : Display
  Display1 : Display
  Divide1 : Product  Inputs=*/
  Divide2 : Product  Inputs=*//
  Initial Capacity(Ah) : Constant  Value=28
  Integrator Limited : Integrator  LimitOutput=on  UpperSaturationLimit=1  LowerSaturationLimit=0
  LoadAh : Scope
  Product : Product
  SOC : Scope
  SOC value : Display
  Scope : Scope
  Scope1 : Scope
  Series RLC Branch : spsSeriesRLCBranchLib/Series RLC Branch  LConnTagsString=__new0  RConnTagsString=__new0  BranchType=R  Resistance=1e-6  Inductance=1e-3  SetiL0=off  InitialCurrent=0  Capacitance=1e-6  Setx0=off  InitialVoltage=0  Measurements=None
  Subsystem : Subsystem
  Subsystem1 : Subsystem
  Sum : Sum  Inputs=|+-
  Sum1 : Sum  Inputs=+--
  Voltage Measurement : spsVoltageMeasurementLib/Voltage Measurement  PhasorSimulation=off  OutputType=Complex  PSBequivalent=0
  battery Temp(k) : Constant  Value=300
  + : PMIOPort  Side=Left
  - : PMIOPort  Port=2  Side=Right
  wires:
  Subsystem/3(R1) -> Divide2/2
  Divide1/1 -> Sum/1
  Product/1 -> Sum1/2
  Current Measurement/1 -> Display1/1, Scope/1, Divide1/1, Product/2, Subsystem1/1(Battery Current)
  Subsystem/1(Em) -> Sum1/1
  battery Temp(k)/1 -> Subsystem1/3(Temp(K)), Subsystem/2(Battery temp)
  Sum/1 -> Integrator Limited/1
  Divide2/1 -> Sum/2
  Subsystem/2(R0) -> Product/1
  Integrator Limited/1 -> Divide2/1, Sum1/3
  Subsystem/4(C1) -> Divide2/3, Divide1/2
  Sum1/1 -> Controlled Voltage Source/1
  Subsystem1/2(SOC) -> Subsystem/1(SOC), SOC value/1, SOC/1
  Subsystem1/1(LoadAh) -> LoadAh/1
  Initial Capacity(Ah)/1 -> Subsystem1/2(InitCap(Ah))
  Voltage Measurement/1 -> Display/1, Scope1/1
  connections:
  Series RLC Branch/RConn1 -- Voltage Measurement/LConn1 -- Current Measurement/LConn1
  Current Measurement/RConn1 -- +/RConn1
  Controlled Voltage Source/LConn1 -- Voltage Measurement/LConn2 -- -/RConn1
  Series RLC Branch/LConn1 -- Controlled Voltage Source/RConn1

== system EV_assigment2/series2/Subsystem10 ==
  Controlled Voltage Source : spsControlledVoltageSourceLib/Controlled Voltage Source  Initialize=on  Source_Type=AC  Amplitude=0  Phase=0  Frequency=0  Measurements=None
  Current Measurement : spsCurrentMeasurementLib/Current Measurement  PhasorSimulation=off  OutputType=Complex  PSBequivalent=0
  Display : Display
  Display1 : Display
  Divide1 : Product  Inputs=*/
  Divide2 : Product  Inputs=*//
  Initial Capacity(Ah) : Constant  Value=28
  Integrator Limited : Integrator  LimitOutput=on  UpperSaturationLimit=1  LowerSaturationLimit=0
  LoadAh : Scope
  Product : Product
  SOC : Scope
  SOC value : Display
  Scope : Scope
  Scope1 : Scope
  Series RLC Branch : spsSeriesRLCBranchLib/Series RLC Branch  LConnTagsString=__new0  RConnTagsString=__new0  BranchType=R  Resistance=1e-6  Inductance=1e-3  SetiL0=off  InitialCurrent=0  Capacitance=1e-6  Setx0=off  InitialVoltage=0  Measurements=None
  Subsystem : Subsystem
  Subsystem1 : Subsystem
  Sum : Sum  Inputs=|+-
  Sum1 : Sum  Inputs=+--
  Voltage Measurement : spsVoltageMeasurementLib/Voltage Measurement  PhasorSimulation=off  OutputType=Complex  PSBequivalent=0
  battery Temp(k) : Constant  Value=300
  + : PMIOPort  Side=Left
  - : PMIOPort  Port=2  Side=Right
  wires:
  Subsystem/3(R1) -> Divide2/2
  Divide1/1 -> Sum/1
  Product/1 -> Sum1/2
  Current Measurement/1 -> Display1/1, Scope/1, Divide1/1, Product/2, Subsystem1/1(Battery Current)
  Subsystem/1(Em) -> Sum1/1
  battery Temp(k)/1 -> Subsystem1/3(Temp(K)), Subsystem/2(Battery temp)
  Sum/1 -> Integrator Limited/1
  Divide2/1 -> Sum/2
  Subsystem/2(R0) -> Product/1
  Integrator Limited/1 -> Divide2/1, Sum1/3
  Subsystem/4(C1) -> Divide2/3, Divide1/2
  Sum1/1 -> Controlled Voltage Source/1
  Subsystem1/2(SOC) -> Subsystem/1(SOC), SOC value/1, SOC/1
  Subsystem1/1(LoadAh) -> LoadAh/1
  Initial Capacity(Ah)/1 -> Subsystem1/2(InitCap(Ah))
  Voltage Measurement/1 -> Display/1, Scope1/1
  connections:
  Series RLC Branch/RConn1 -- Voltage Measurement/LConn1 -- Current Measurement/LConn1
  Current Measurement/RConn1 -- +/RConn1
  Controlled Voltage Source/LConn1 -- Voltage Measurement/LConn2 -- -/RConn1
  Series RLC Branch/LConn1 -- Controlled Voltage Source/RConn1

== system EV_assigment2/series2/Subsystem11 ==
  Controlled Voltage Source : spsControlledVoltageSourceLib/Controlled Voltage Source  Initialize=on  Source_Type=AC  Amplitude=0  Phase=0  Frequency=0  Measurements=None
  Current Measurement : spsCurrentMeasurementLib/Current Measurement  PhasorSimulation=off  OutputType=Complex  PSBequivalent=0
  Display : Display
  Display1 : Display
  Divide1 : Product  Inputs=*/
  Divide2 : Product  Inputs=*//
  Initial Capacity(Ah) : Constant  Value=28
  Integrator Limited : Integrator  LimitOutput=on  UpperSaturationLimit=1  LowerSaturationLimit=0
  LoadAh : Scope
  Product : Product
  SOC : Scope
  SOC value : Display
  Scope : Scope
  Scope1 : Scope
  Series RLC Branch : spsSeriesRLCBranchLib/Series RLC Branch  LConnTagsString=__new0  RConnTagsString=__new0  BranchType=R  Resistance=1e-6  Inductance=1e-3  SetiL0=off  InitialCurrent=0  Capacitance=1e-6  Setx0=off  InitialVoltage=0  Measurements=None
  Subsystem : Subsystem
  Subsystem1 : Subsystem
  Sum : Sum  Inputs=|+-
  Sum1 : Sum  Inputs=+--
  Voltage Measurement : spsVoltageMeasurementLib/Voltage Measurement  PhasorSimulation=off  OutputType=Complex  PSBequivalent=0
  battery Temp(k) : Constant  Value=300
  + : PMIOPort  Side=Left
  - : PMIOPort  Port=2  Side=Right
  wires:
  Subsystem/3(R1) -> Divide2/2
  Divide1/1 -> Sum/1
  Product/1 -> Sum1/2
  Current Measurement/1 -> Display1/1, Scope/1, Divide1/1, Product/2, Subsystem1/1(Battery Current)
  Subsystem/1(Em) -> Sum1/1
  battery Temp(k)/1 -> Subsystem1/3(Temp(K)), Subsystem/2(Battery temp)
  Sum/1 -> Integrator Limited/1
  Divide2/1 -> Sum/2
  Subsystem/2(R0) -> Product/1
  Integrator Limited/1 -> Divide2/1, Sum1/3
  Subsystem/4(C1) -> Divide2/3, Divide1/2
  Sum1/1 -> Controlled Voltage Source/1
  Subsystem1/2(SOC) -> Subsystem/1(SOC), SOC value/1, SOC/1
  Subsystem1/1(LoadAh) -> LoadAh/1
  Initial Capacity(Ah)/1 -> Subsystem1/2(InitCap(Ah))
  Voltage Measurement/1 -> Display/1, Scope1/1
  connections:
  Series RLC Branch/RConn1 -- Voltage Measurement/LConn1 -- Current Measurement/LConn1
  Current Measurement/RConn1 -- +/RConn1
  Controlled Voltage Source/LConn1 -- Voltage Measurement/LConn2 -- -/RConn1
  Series RLC Branch/LConn1 -- Controlled Voltage Source/RConn1

== system EV_assigment2/series2/Subsystem12 ==
  Controlled Voltage Source : spsControlledVoltageSourceLib/Controlled Voltage Source  Initialize=on  Source_Type=AC  Amplitude=0  Phase=0  Frequency=0  Measurements=None
  Current Measurement : spsCurrentMeasurementLib/Current Measurement  PhasorSimulation=off  OutputType=Complex  PSBequivalent=0
  Display : Display
  Display1 : Display
  Divide1 : Product  Inputs=*/
  Divide2 : Product  Inputs=*//
  Initial Capacity(Ah) : Constant  Value=28
  Integrator Limited : Integrator  LimitOutput=on  UpperSaturationLimit=1  LowerSaturationLimit=0
  LoadAh : Scope
  Product : Product
  SOC : Scope
  SOC value : Display
  Scope : Scope
  Scope1 : Scope
  Series RLC Branch : spsSeriesRLCBranchLib/Series RLC Branch  LConnTagsString=__new0  RConnTagsString=__new0  BranchType=R  Resistance=1e-6  Inductance=1e-3  SetiL0=off  InitialCurrent=0  Capacitance=1e-6  Setx0=off  InitialVoltage=0  Measurements=None
  Subsystem : Subsystem
  Subsystem1 : Subsystem
  Sum : Sum  Inputs=|+-
  Sum1 : Sum  Inputs=+--
  Voltage Measurement : spsVoltageMeasurementLib/Voltage Measurement  PhasorSimulation=off  OutputType=Complex  PSBequivalent=0
  battery Temp(k) : Constant  Value=300
  + : PMIOPort  Side=Left
  - : PMIOPort  Port=2  Side=Right
  wires:
  Subsystem/3(R1) -> Divide2/2
  Divide1/1 -> Sum/1
  Product/1 -> Sum1/2
  Current Measurement/1 -> Display1/1, Scope/1, Divide1/1, Product/2, Subsystem1/1(Battery Current)
  Subsystem/1(Em) -> Sum1/1
  battery Temp(k)/1 -> Subsystem1/3(Temp(K)), Subsystem/2(Battery temp)
  Sum/1 -> Integrator Limited/1
  Divide2/1 -> Sum/2
  Subsystem/2(R0) -> Product/1
  Integrator Limited/1 -> Divide2/1, Sum1/3
  Subsystem/4(C1) -> Divide2/3, Divide1/2
  Sum1/1 -> Controlled Voltage Source/1
  Subsystem1/2(SOC) -> Subsystem/1(SOC), SOC value/1, SOC/1
  Subsystem1/1(LoadAh) -> LoadAh/1
  Initial Capacity(Ah)/1 -> Subsystem1/2(InitCap(Ah))
  Voltage Measurement/1 -> Display/1, Scope1/1
  connections:
  Series RLC Branch/RConn1 -- Voltage Measurement/LConn1 -- Current Measurement/LConn1
  Current Measurement/RConn1 -- +/RConn1
  Controlled Voltage Source/LConn1 -- Voltage Measurement/LConn2 -- -/RConn1
  Series RLC Branch/LConn1 -- Controlled Voltage Source/RConn1
